simulink model "D_Axis"  (R2024b)
settings: Solver=VariableStepAuto  StartTime=0.0  StopTime=t(end)  RelTol=1e-3
values from neighbouring files (symbols this model uses):
  Lq = 2.47478e-3    (= 0.00247478)    [main.m]
libraries: cstblocks x2
settings Model: Creator=mushen  LastModifiedBy=mushen

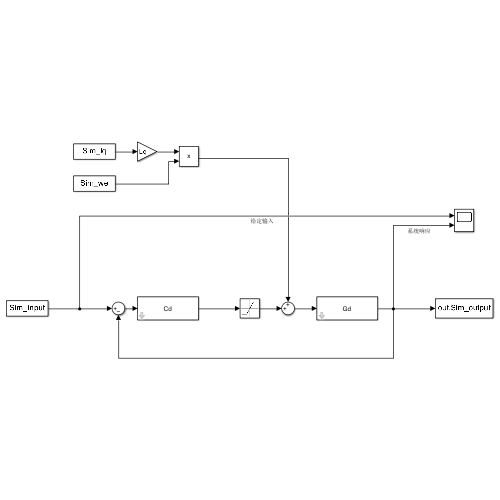
[thumbnail: Simulink's stored preview of the top-level diagram]
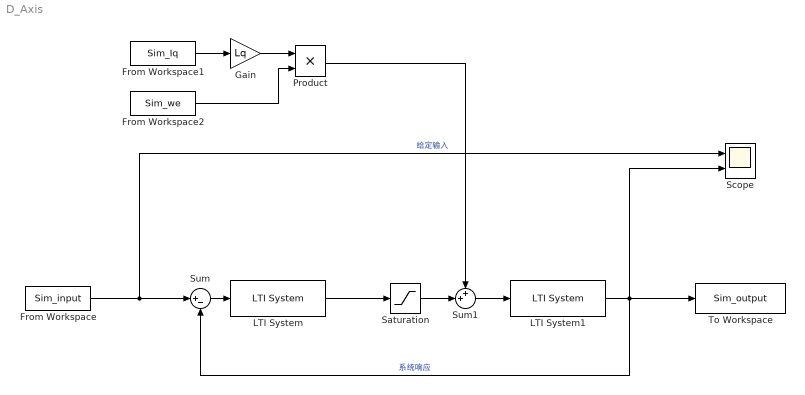
== system D_Axis ==
  From Workspace : FromWorkspace  VariableName=Sim_input
  From Workspace1 : FromWorkspace  VariableName=Sim_Iq
  From Workspace2 : FromWorkspace  VariableName=Sim_we
  Gain : Gain  Gain=Lq
  LTI System : cstblocks/LTI System  sys=Cd  IC=[]  PadeOrder=0
  LTI System1 : cstblocks/LTI System  sys=Gd  IC=[]  PadeOrder=1
  Product : Product
  Saturation : Saturate  UpperLimit=12/sqrt(3)  LowerLimit=-12/sqrt(3)
  Scope : Scope  NumInputPorts=2
  Sum : Sum  Inputs=|+-
  Sum1 : Sum  Inputs=++|
  To Workspace : ToWorkspace  VariableName=Sim_output  SaveFormat=Timeseries  SampleTime=-1
  wires:
  Sum/1 -> LTI System/1
  LTI System1/1 -> Scope/2, To Workspace/1, Sum/2  "系统响应"
  From Workspace/1 -> Scope/1, Sum/1  "给定输入"
  LTI System/1 -> Saturation/1
  From Workspace1/1 -> Gain/1
  Gain/1 -> Product/1
  From Workspace2/1 -> Product/2
  Product/1 -> Sum1/1
  Saturation/1 -> Sum1/2
  Sum1/1 -> LTI System1/1
